simulink model "bpsk_rx1_8"  (Simulink 9.3)
settings: Solver=FixedStepDiscrete  StartTime=0.0  StopTime=2000  RelTol=1e-3
undefined symbols (not defined in the file): input_stream_sample
libraries: dsp_blocks x9, simulink x1
settings Model: Creator=dell  LastModifiedBy=dell
settings DataIOCC: SaveFormat=Dataset  SignalLoggingSaveFormat=Dataset  ReturnWorkspaceOutputs=on
settings OptimizationCC: LifeSpan=auto
settings DebuggingCC: UnderspecifiedInitializationDetection=Simplified  MergeDetectMultiDrivingBlocksExec=error  FcnCallInpInsideContextMsg=error  SFUnexpectedBacktrackingDiag=error  SFNoUnconditionalDefaultTransitionDiag=error  SFExecutionAtInitializationDiag=warning  ArithmeticOperatorsInVariantConditions=error
settings HardwareCC: ProdBitPerPointer=64  ProdBitPerSizeT=64  ProdBitPerPtrDiffT=64  ProdLargestAtomicFloat=Float  ProdIntDivRoundTo=Zero  ProdEndianess=LittleEndian  ProdWordSize=64  ProdHWDeviceType=Intel->x86-64 (Windows64)
settings ModelReferenceCC: PropagateSignalLabelsOutOfModel=on
settings SFSimCC: SimUseLocalCustomCode=on
settings RTWCC: RTWUseLocalCustomCode=on
settings CodeAppCC: StateflowObjectComments=off
settings GRTTargetCC: TargetLangStandard=C99 (ISO)  CombineOutputUpdateFcns=on  GRTInterface=off
settings ConfigComp: CovMetricSettings=dwe  CovHtmlReporting=off  CovSaveCumulativeToWorkspaceVar=off  CovSaveSingleToWorkspaceVar=off  CovExternalEMLEnable=on

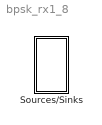
== system bpsk_rx1_8 ==
  Sources/Sinks : Subsystem  AncestorBlock=dsp_blocks/Sources//Sinks

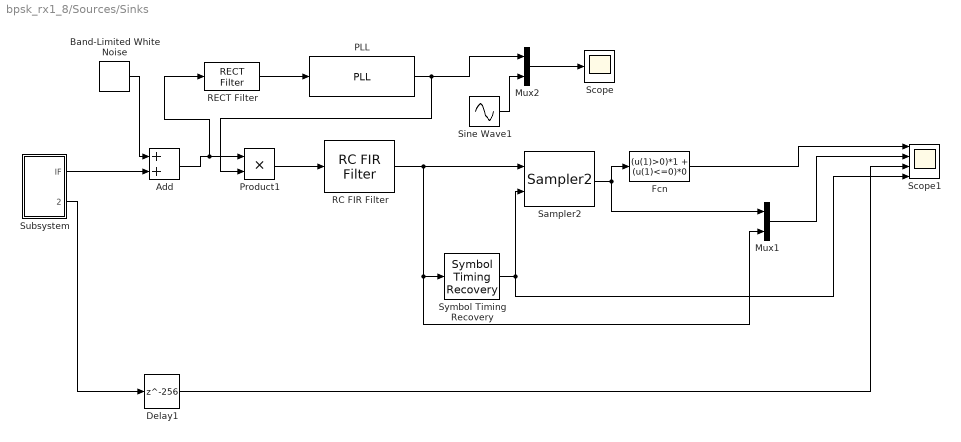
== system bpsk_rx1_8/Sources/Sinks ==
  Add : Sum
  Band-Limited White Noise : simulink/Sources/Band-Limited White Noise  Cov=[0.01]  Ts=1  seed=[23341]
  Delay1 : Delay  DelayLength=256
  Fcn : Fcn  Expr=(u(1)>0)*1 + (u(1)<=0)*0
  Mux1 : Mux  Inputs=2
  Mux2 : Mux  Inputs=2
  PLL : dsp_blocks/Timing /PLL  freq=0.05  freq_out=0.1  phi=0  amp=2  xi=1  K=2  T=200
  Product1 : Product
  RC FIR Filter : dsp_blocks/Filters/RC FIR Filter  period=50  beta=0.5  root=on  filt_len=512  win_type=on
  RECT Filter : dsp_blocks/Filters/RECT Filter  f0=0.03  f1=0.07  filt_len=80
  Sampler2 : dsp_blocks/Conversions/Sampler2
  Scope : Scope
  Scope1 : Scope  NumInputPorts=4
  Sine Wave1 : Sin  Amplitude=2  Frequency=2*pi*0.1  SampleTime=0
  Subsystem : Subsystem
  Symbol Timing Recovery : dsp_blocks/Timing /Symbol Timing Recovery  T=50  Tl=10000  tadj=-1
  wires:
  PLL/1 -> Product1/2, Mux2/1
  Subsystem/2("Debug ") -> Delay1/1
  Delay1/1 -> Scope1/3
  Product1/1 -> RC FIR Filter/1
  RC FIR Filter/1 -> Symbol Timing Recovery/1, Mux1/2, Sampler2/1
  Sampler2/1 -> Fcn/1, Mux1/1
  Fcn/1 -> Scope1/1
  Mux1/1 -> Scope1/2
  RECT Filter/1 -> PLL/1
  Sine Wave1/1 -> Mux2/2
  Mux2/1 -> Scope/1
  Symbol Timing Recovery/1 -> Sampler2/2, Scope1/4
  Band-Limited White Noise/1 -> Add/1
  Subsystem/1(IF) -> Add/2
  Add/1 -> RECT Filter/1, Product1/1

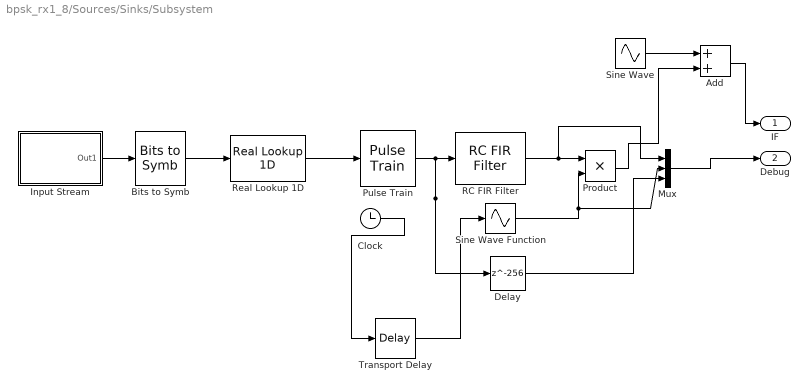
== system bpsk_rx1_8/Sources/Sinks/Subsystem ==
  Add : Sum
  Bits to Symb : dsp_blocks/Conversions/Bits to Symb
  Clock : Clock
  Delay : Delay  DelayLength=256
  Input Stream : Subsystem  mask{period=50, width=1, fname=rand.mat}
      mask prompts: fname "Data Filename"
      mask help: Input Stream: Reads binary data from an input file. Outputs a new value once per period. Width allows you to multiplex output.
      mask init:
      | load(fname); N = floor(length(data)/width); data = reshape(data(1:N*width),width,N);
      mask Help: The function loads the binary data from file fname, which should have a single vector called "data".  The output of the block is updated once every T=width*period.
      mask Display: disp(sprintf('file=%s\nT=%g w=%d', fname, period, width))
  Mux : Mux  Inputs=3
  Product : Product
  Pulse Train : dsp_blocks/Conversions/Pulse Train  period=50
  RC FIR Filter : dsp_blocks/Filters/RC FIR Filter  period=50  beta=0.5  root=on  filt_len=512  win_type=on
  Real Lookup 1D : dsp_blocks/Conversions/Real Lookup 1D  table=[-1 1]
  Sine Wave : Sin  Amplitude=0.05  Frequency=2*pi*0.05  SampleTime=0
  Sine Wave Function : Sin  TimeSource=Use external signal  Frequency=2*pi*0.1  SampleTime=0
  Transport Delay : TransportDelay
  IF : Outport
  "Debug " : Outport  Port=2
  wires:
  Delay/1 -> Mux/3
  RC FIR Filter/1 -> Mux/1, Product/1
  Mux/1 -> "Debug "/1
  Sine Wave Function/1 -> Mux/2, Product/2
  Input Stream/1(Out1) -> Bits to Symb/1
  Bits to Symb/1 -> Real Lookup 1D/1
  Real Lookup 1D/1 -> Pulse Train/1
  Pulse Train/1 -> Delay/1, RC FIR Filter/1
  Clock/1 -> Transport Delay/1
  Transport Delay/1 -> Sine Wave Function/1
  Sine Wave/1 -> Add/1
  Product/1 -> Add/2
  Add/1 -> IF/1

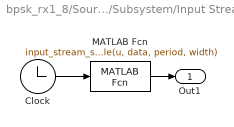
== system bpsk_rx1_8/Sources/Sinks/Subsystem/Input Stream ==
  Clock : Clock
  MATLAB Fcn : MATLABFcn  MATLABFcn=input_stream_sample(u, data, period, width)  OutputDimensions=width  Output1D=off
  Out1 : Outport
  wires:
  Clock/1 -> MATLAB Fcn/1
  MATLAB Fcn/1 -> Out1/1
